simulink model "AMR_main_24a_TesteMobotic"  (R2024a)
settings: Solver=FixedStepAuto  StartTime=0.0  StopTime=inf  FixedStep=1e-3  RelTol=1e-3
model workspace (MAT data in the model file):
  RTK_health_condition = 30
  mdlWSDbList = ["tramontina_database_curtis.dbc" "tramontina_database_mobotic.dbc" "tramontina_database_nvidia.dbc" "tramontina_database_sick_modbus.dbc" "tramontina_database_xsens.dbc"]
undefined symbols (not defined in the file or in its folder): Down, Pull
libraries: tramontina_database_nvidialib x11, speedgoatlib_IO60X_IO69X x10, tramontina_database_curtislib x7, tramontina_database_xsenslib x4, tramontina_database_moboticlib x2, speedgoatlib_IO691 x2, canmsglib x1
(part 1 of 2)
settings Model: DataDictionary=configuration_dictionary.sldd  SimulationMode=external  ExtModeEnableFloating=off  ExtModeTrigDuration=100000  Creator=matlab.cut  LastModifiedBy=matlab.cut
settings SolverCC: ConcurrentTasks=on  PositivePriorityOrder=on
settings OptimizationCC: BlockReduction=off  DefaultParameterBehavior=Inlined  OptimizeBlockIOStorage=off  EnhancedBackFolding=on  PassReuseOutputArgsThreshold=0  OptimizeBlockOrder=speed  DifferentSizesBufferReuse=on
settings DebuggingCC: UnderspecifiedInitializationDetection=Classic  MergeDetectMultiDrivingBlocksExec=none  TasksWithSamePriorityMsg=none  ParameterTunabilityLossMsg=error
settings HardwareCC: ProdBitPerLong=64  ProdLongLongMode=on  ProdHWDeviceType=Intel->x86-64 (Linux 64)
settings ModelReferenceCC: PropagateSignalLabelsOutOfModel=off
settings SFSimCC: MATLABDynamicMemAlloc=off
settings RTWCC: Description=Speedgoat Real-Time Target Machine  SystemTargetFile=speedgoat.tlc  TemplateMakefile=slrealtime_default_tmf  Toolchain=Simulink Real-Time Toolchain  BuildConfiguration=Faster Runs  CodeExecutionProfiling=on  TargetLang=C++  GPUComputeCapability=3.5
settings CodeAppCC: ForceParamTrailComments=on  MaxIdLength=127  OperatorAnnotations=on
settings SimulinkRealTimeTargetCC: InstructionSetFMA=off  LogToMDFFile=off

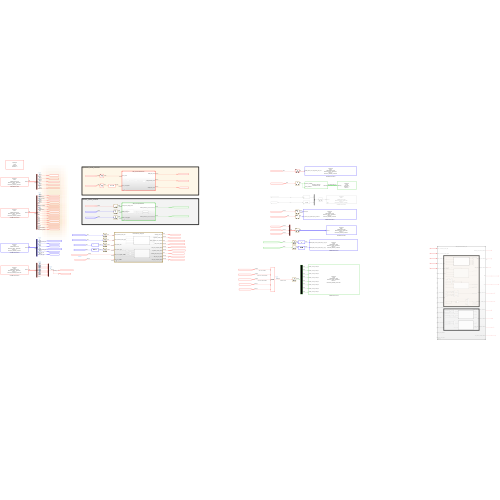
[thumbnail: Simulink's stored preview of the top-level diagram]
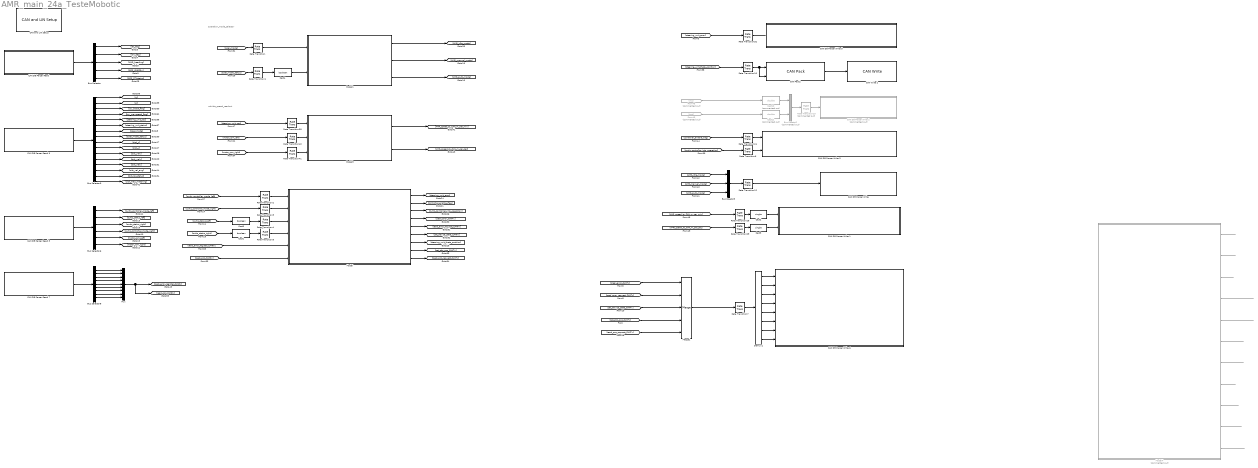
== system AMR_main_24a_TesteMobotic ==
  note: operation_mode_selector
  note: vehicle_speed_readout
  Bus Creator2 : BusCreator  Commented=on  Inputs=2
  Bus Creator3 : BusCreator  Inputs=3
  Bus Selector : BusSelector  OutputSignals=ID113_LongLat.latitude,ID113_LongLat.longitude,ID34_EulerAngles.yaw,ID17_StatusWord.GNSSfix,ID17_StatusWord.RtkStatus
  Bus Selector6 : BusSelector  OutputSignals=ID1830_controller_status_left.controller_mode_left,ID1830_controller_status_left.MessageStatus.Status,ID1831_controller_status_right.MessageStatus.Status,ID1831_controller_status_right.controller_mode_right,ID422_curtis_feedback_message_left.motor_rpm_left,ID423_curtis_feedback_message_right.motor_rpm_right
  Bus Selector8 : BusSelector  OutputSignals=ID1459_feedback_word.MessageStatus.Status,ID1459_feedback_word.byte0,ID1459_feedback_word.byte1,ID1459_feedback_word.byte2,ID1459_feedback_word.byte3,ID1459_feedback_word.byte4,ID1459_feedback_word.byte5,ID1459_feedback_word.byte6,ID1459_feedback_word.byte7
  Bus Selector9 : BusSelector  OutputSignals=ID368_joystick_axes.joystick_throttle,ID368_joystick_axes.joystick_direction,ID369_joystick_buttons.button_5,ID369_joystick_buttons.button_6,ID288_mobotic_feedback_pos.position_feedback,ID288_mobotic_feedback_pos.MessageStatus.Status,ID343_AMR_OperationMode.OperationMode,ID343_AMR_OperationMode.MessageStatus.Status,ID370_outdoor_scanner_PosX.X,ID371_outdoor_scanner_PosY.Y,ID372_outdoor_scanner_Yaw_Status.Yaw,ID373_outdoor_scanner_Odometer_Vel.velX,ID373_outdoor_scanner_Odometer_Vel.velY,ID373_outdoor_scanner_Odometer_Vel.velAng,ID372_outdoor_scanner_Yaw_Status.LocalizationStatus,ID372_outdoor_scanner_Yaw_Status.MapMatchingStatus
  CAN DB Parser Read : Subsystem
      settings: OpenFcn=sg_can.OpenFcnRead;
      mask Help: eval('sg.utils.help.show(''io_main/refentry_ref_can_ofa_parsing_read'');')
      mask Display: disp('Speedgoat\nIO691\nCAN DB Parser Read\nModule ID: IO691 - Module ID 1\nChannel:  1\ntramontina_database_xsens.dbc ');
  CAN DB Parser Read 3 : Subsystem
      settings: OpenFcn=sg_can.OpenFcnRead;
      mask Help: eval('sg.utils.help.show(''io_main/refentry_ref_can_ofa_parsing_read'');')
      mask Display: disp('Speedgoat\nIO691\nCAN DB Parser Read\nModule ID: IO691 - Module ID 1\nChannel:  1\ntramontina_database_curtis.dbc ');
  CAN DB Parser Read 7 : Subsystem
      settings: OpenFcn=sg_can.OpenFcnRead;
      mask Help: eval('sg.utils.help.show(''io_main/refentry_ref_can_ofa_parsing_read'');')
      mask Display: disp('Speedgoat\nIO691\nCAN DB Parser Read\nModule ID: IO691 - Module ID 1\nChannel:  1\ntramontina_database_mobotic.dbc ');
  CAN DB Parser Read 9 : Subsystem
      settings: OpenFcn=sg_can.OpenFcnRead;
      mask Help: eval('sg.utils.help.show(''io_main/refentry_ref_can_ofa_parsing_read'');')
      mask Display: disp('Speedgoat\nIO691\nCAN DB Parser Read\nModule ID: IO691 - Module ID 1\nChannel:  1\ntramontina_database_nvidia.dbc ');
  "CAN DB Parser Write " : Subsystem
      settings: OpenFcn=sg_can.OpenFcnWrite;
      mask Help: eval('sg.utils.help.show(''io_main/refentry_ref_can_ofa_parsing_write'');')
      mask Display: disp('Speedgoat\nIO691\nCAN DB Parser Write\nModule ID: IO691 - Module ID 1\nChannel:  1\ntramontina_database_nvidia.dbc ');
  CAN DB Parser Write 1 : Subsystem
      settings: OpenFcn=sg_can.OpenFcnWrite;
      mask Help: eval('sg.utils.help.show(''io_main/refentry_ref_can_ofa_parsing_write'');')
      mask Display: disp('Speedgoat\nIO691\nCAN DB Parser Write\nModule ID: IO691 - Module ID 1\nChannel:  1\ntramontina_database_nvidia.dbc ');
  CAN DB Parser Write 2 : Subsystem  Commented=on
      settings: OpenFcn=sg_can.OpenFcnWrite;
      mask Help: eval('sg.utils.help.show(''io_main/refentry_ref_can_ofa_parsing_write'');')
      mask Display: disp('Speedgoat\nIO691\nCAN DB Parser Write\nModule ID: IO691 - Module ID 1\nChannel:  1\ntramontina_database_curtis.dbc ');
  CAN DB Parser Write 3 : Subsystem
      settings: OpenFcn=sg_can.OpenFcnWrite;
      mask Help: eval('sg.utils.help.show(''io_main/refentry_ref_can_ofa_parsing_write'');')
      mask Display: disp('Speedgoat\nIO691\nCAN DB Parser Write\nModule ID: IO691 - Module ID 1\nChannel:  1\ntramontina_database_curtis.dbc ');
  CAN DB Parser Write 5 : Subsystem
      settings: OpenFcn=sg_can.OpenFcnWrite;
      mask Help: eval('sg.utils.help.show(''io_main/refentry_ref_can_ofa_parsing_write'');')
      mask Display: disp('Speedgoat\nIO691\nCAN DB Parser Write\nModule ID: IO691 - Module ID 1\nChannel:  1\ntramontina_database_nvidia.dbc ');
  CAN DB Parser Write 6 : Subsystem
      settings: OpenFcn=sg_can.OpenFcnWrite;
      mask Help: eval('sg.utils.help.show(''io_main/refentry_ref_can_ofa_parsing_write'');')
      mask Display: disp('Speedgoat\nIO691\nCAN DB Parser Write\nModule ID: IO691 - Module ID 1\nChannel:  1\ntramontina_database_mobotic.dbc ');
  CAN Pack2 : canmsglib/CAN Pack  MsgList=(none)  MsgName=CAN Msg  MsgIDType=Standard (11-bit identifier)  MsgIdentifier=0x120  MsgLength=8  Remote=off  ApplyMinMax=off  BusOutput=on  SignalInfo={ 'position_feedback', '0', '32', 'LE', 'signed', 'Standard', '0', '1', '0', '-inf', 'inf'; 'pulse_feedback', '32', '32', 'LE', 'signed', 'Standard', '0', '1', '0', '-Inf', 'Inf' }
      settings: DataFormat=manually specified signals
  CAN Write 2 : speedgoatlib_IO691/CAN Write   moduleType=IO691  id=1  channel=1  canType=CAN (HS)  messageType=CAN (HS)  useBusIn=on  numOfMsg=1  enableInput=off  enableStatusPort=off  ts=10e-3  initValues=[691 1 0.01 0 1 1 0 1 0 1]
      settings: SourceProductName=IO691
  "CAN and LIN Setup " : speedgoatlib_IO691/CAN and LIN Setup   moduleInitValues="[691    1    1   -1   -1]"  id=1  moduleType=IO691  pciSlot=-1  canChn1=CAN (HS)  canChn2=Disabled  canChn3=Disabled  canChn4=Disabled  linChn1=Disabled  linChn2=Disabled  canInitStructArray=[]  canTermStructArray=[]  gpioChnx=Disabled  canChn1InitValues="[2   2   8   1  16   3  19   2   2   5   2   0]"  arbBdrChn1=500 kBaud  clockDividerChn1=Enable  arbManBdrChn1=[8,1,16,3]  fdBdrChn1=5.0 MBaud  fdManBdrChn1=[2,2,5,2]  termResistor1=off  canChn2InitValues="[1   0   2   8  31   8  19   2   2   5   2   0]"  arbBdrChn2=1.0 MBaud  clockDividerChn2=Enable  arbManBdrChn2=[2,8,31,8]  fdBdrChn2=5.0 MBaud  fdManBdrChn2=[2,2,5,2]  termResistor2=off  canChn3InitValues="[1   0   2   8  31   8  19   2   2   5   2   0]"  arbBdrChn3=1.0 MBaud  clockDividerChn3=Enable  arbManBdrChn3=[2,8,31,8]  fdBdrChn3=5.0 MBaud  fdManBdrChn3=[2,2,5,2]  termResistor3=off  canChn4InitValues="[1   0   2   8  31   8  19   2   2   5   2   0]"  arbBdrChn4=1.0 MBaud  clockDividerChn4=Enable  arbManBdrChn4=[2,8,31,8]  fdBdrChn4=5.0 MBaud  fdManBdrChn4=[2,2,5,2]  termResistor4=off  linChn1InitValues="[0  9600]"  linBtrChn1=9600  linChn2InitValues="[0  9600]"  linBtrChn2=9600  doInitTermStruct="[0  5  0  0  0]"  parDoChannels=[1 2]  parDoVoltage=5  parDoInitValues=0  parDoReset=1  parNumOfDoS=0  parDiChannels=[3 4]  parDiVoltage=5  parDiPull=Pull-Down
      settings: LibrarySourceBlock=speedgoatlib_IO602_IO691/CAN and LIN Setup
  Cast1 : DataTypeConversion  OutDataTypeStr=boolean  SaturateOnIntegerOverflow=off  RndMeth=Floor
  Cast10 : DataTypeConversion  Commented=on  OutDataTypeStr=double  SaturateOnIntegerOverflow=off  RndMeth=Floor
  Cast11 : DataTypeConversion  Commented=on  OutDataTypeStr=double  SaturateOnIntegerOverflow=off  RndMeth=Floor
  Cast2 : DataTypeConversion  OutDataTypeStr=single  SaturateOnIntegerOverflow=off  RndMeth=Floor
  Cast3 : DataTypeConversion  OutDataTypeStr=single  SaturateOnIntegerOverflow=off  RndMeth=Floor
  Cast4 : DataTypeConversion  OutDataTypeStr=boolean  SaturateOnIntegerOverflow=off  RndMeth=Floor
  Cast5 : DataTypeConversion  OutDataTypeStr=boolean  SaturateOnIntegerOverflow=off  RndMeth=Floor
  Demux1 : Demux  Outputs=8
  From43 : From  Commented=on  GotoTag=rws
  From45 : From  Commented=on  GotoTag=lws
  Merge1 : Merge  Inputs=5
  Model : ModelReference  ModelNameDialog=MoboticStartup_TimingSync.slx  SimulationMode=Normal  ModelReferenceVersion=1.12
  Model1 : ModelReference  ModelNameDialog=AMR_OperationModeSelector.slx  SimulationMode=Normal  ModelReferenceVersion=2.2
  Model3 : ModelReference  ModelNameDialog=AMR_VehicleSpeedReadout.slx  SimulationMode=Normal  ModelReferenceVersion=2.1
  Model4 : ModelReference  Commented=on  ModelNameDialog=AMR_MotorControlUnit_23b.slx  SimulationMode=Normal  ModelReferenceVersion=2.8
  Mux : Mux  Inputs=9
  Rate Transition{,1..7,10,24,28..29,32,38,40..41} (16 alike) : RateTransition
  Rate Transition12 : RateTransition  Deterministic=off
  Rate Transition15 : RateTransition  Commented=on
  wires:
  Rate Transition32/1 -> ?
  Rate Transition28/1 -> Cast2/1
  [AMR_speed_to_CAN_m_per_sec] -> Rate Transition29/1
  [AMR_speed_to_CAN_m_per_min] -> Rate Transition28/1
  CAN Pack2/1 -> CAN Write 2/1
  Bus Creator2/1 -> Rate Transition15/1
  From43/1 -> Cast11/1  "rws"
  Cast10/1 -> Bus Creator2/1
  Rate Transition6/1 -> CAN DB Parser Write 3/2(ID0_curtis_input_operational.pre_operational)
  Bus Creator3/1 -> Rate Transition12/1
  [steering_unit_error] -> Rate Transition32/1
  Rate Transition10/1 -> CAN Pack2/2, CAN Pack2/1
  Rate Transition29/1 -> Cast3/1
  [curtis_controller_into_operation] -> Rate Transition6/1
  From45/1 -> Cast10/1  "lws"
  Cast11/1 -> Bus Creator2/2
  [steering_unit_theta_position] -> Rate Transition10/1
  [controller_enable_flag] -> Rate Transition24/1
  Rate Transition15/1 -> CAN DB Parser Write 2/1(CAN Tx)
  Rate Transition24/1 -> CAN DB Parser Write 3/1(Enable Input)
  [oper_mode] -> Rate Transition/1
  Cast4/1 -> Model1/2
  Model1/1 -> [AMR_idle_mode]
  Model1/2 -> [AMR_manual_mode]
  Model1/3 -> [AMR_auto_mode]
  ? -> Model4/3
  ? -> Model4/1
  ? -> Model4/4
  ? -> Model4/2
  [motor_rpm_right] -> Rate Transition41/1
  [steering_unit_pos] -> Rate Transition38/1
  [motor_rpm_left] -> Rate Transition40/1
  Model3/1 -> [AMR_speed_to_CAN_m_per_min]
  Model3/2 -> [AMR_speed_to_CAN_m_per_sec]
  Rate Transition38/1 -> Model3/1
  Rate Transition41/1 -> Model3/3
  Rate Transition40/1 -> Model3/2
  Cast2/1 -> CAN DB Parser Write 1/1(ID290_AMR_vehicle_speed.speed_m_per_min)
  Cast3/1 -> CAN DB Parser Write 1/2(ID290_AMR_vehicle_speed.speed_m_per_s)
  [oper_mode_status] -> Rate Transition1/1
  [AMR_idle_mode] -> Bus Creator3/1
  [AMR_auto_mode] -> Bus Creator3/3
  [AMR_manual_mode] -> Bus Creator3/2
  Rate Transition12/1 -> "CAN DB Parser Write "/1(CAN Tx)
  Rate Transition/1 -> Model1/1
  Rate Transition1/1 -> Cast4/1
  Model4/1 -> ?
  Model4/5 -> ?
  Model4/4 -> ?
  Model4/6 -> ?
  Model4/7 -> ?
  Model4/8 -> ?
  Model4/2 -> ?  "lws"
  Model4/3 -> ?  "rws"
  Model4/9 -> ?
  Model4/10 -> ?
  Model4/11 -> ?
  Bus Selector/1 -> [lat_deg]  "<latitude>"
  Bus Selector6/2 -> [curtis_status_left]  "<Status>"
  Bus Selector9/8 -> [oper_mode_status]  "<Status>"
  Bus Selector9/7 -> [oper_mode]  "<OperationMode>"
  Bus Selector9/3 -> [joy_boost_flag]  "<button_5>"
  Bus Selector9/1 -> [xj]  "<joystick_throttle>"
  Bus Selector9/4 -> [joy_maxspeed_flag]  "<button_6>"
  Bus Selector/4 -> [GPS_GNSSfix]  "<GNSSfix>"
  Bus Selector9/2 -> [yj]  "<joystick_direction>"
  Bus Selector8/7 -> Mux/7  "<byte5>"
  CAN DB Parser Read 9/1(CAN Rx) -> Bus Selector9/1
  Bus Selector8/5 -> Mux/5  "<byte3>"
  Bus Selector9/13 -> [sick_vely]  "<velY>"
  Bus Selector8/1 -> Mux/1  "<Status>"
  Bus Selector9/5 -> [steering_unit_pos]  "<position_feedback>"
  Bus Selector8/2 -> Mux/2  "<byte0>"
  CAN DB Parser Read 3/1(CAN Rx) -> Bus Selector6/1
  Bus Selector9/9 -> [sick_x]  "<X>"
  CAN DB Parser Read 7/1(CAN Rx) -> Bus Selector8/1
  Bus Selector8/3 -> Mux/3  "<byte1>"
  Bus Selector8/6 -> Mux/6  "<byte4>"
  Mux/1 -> [read_pos_CANRx], [read_error_register_CANRx]  "mobotic_Rx"
  Bus Selector8/8 -> Mux/8  "<byte6>"
  Bus Selector8/9 -> Mux/9  "<byte7>"
  Bus Selector6/4 -> [curtis_controller_mode_right]  "<controller_mode_right>"
  Bus Selector9/10 -> [sick_y]  "<Y>"
  Bus Selector9/16 -> [sick_map_matching]  "<MapMatchingStatus>"
  Bus Selector9/12 -> [sick_velx]  "<velX>"
  Bus Selector9/15 -> [sick_loc_status]  "<LocalizationStatus>"
  Bus Selector/5 -> [GPS_RTKstatus]  "<RtkStatus>"
  Bus Selector9/14 -> [sick_vel_ang]  "<velAng>"
  Bus Selector9/6 -> [steering_unit_status]  "<Status>"
  Bus Selector6/5 -> [motor_rpm_left]  "<motor_rpm_left>"
  Bus Selector9/11 -> [sick_yaw]  "<Yaw>"
  Bus Selector6/6 -> [motor_rpm_right]  "<motor_rpm_right>"
  Bus Selector/3 -> [AMR_heading]  "<yaw>"
  Bus Selector6/3 -> [curtis_status_right]  "<Status>"
  Bus Selector8/4 -> Mux/4  "<byte2>"
  Bus Selector6/1 -> [curtis_controller_mode_left]  "<controller_mode_left>"
  CAN DB Parser Read/1(CAN Rx) -> Bus Selector/1
  Bus Selector/2 -> [lon_deg]  "<longitude>"
  ? -> Model4/5
  [curtis_controller_mode_left] -> Rate Transition2/1
  Cast5/1 -> Rate Transition4/1
  Cast1/1 -> Rate Transition5/1
  [curtis_controller_mode_right] -> Rate Transition3/1
  [curtis_status_left] -> Cast5/1
  [curtis_status_right] -> Cast1/1
  [read_error_register_CANRx] -> Model/5
  [read_pos_CANRx] -> Model/6
  Model/9 -> [read_pos_request_CANTx]
  Model/8 -> [set_abs_pos_CANTx]
  Model/7 -> [steering_unit_theta_position]
  Model/5 -> [read_error_request_CANTx]
  Model/6 -> [set_device_state_CANTx]
  Model/4 -> [clear_error_CANTx]
  Model/3 -> [curtis_controller_into_operation]
  Model/2 -> [controller_enable_flag]
  Model/1 -> [steering_unit_error]
  [clear_error_CANTx] -> Merge1/1  "clear_error_CANTx"
  Merge1/1 -> Rate Transition7/1  "mobotic_merge"
  [read_error_request_CANTx] -> Merge1/2  "read_error_request_CANTx"
  [set_device_state_CANTx] -> Merge1/3  "set_device_state_CANTx"
  [set_abs_pos_CANTx] -> Merge1/4
  [read_pos_request_CANTx] -> Merge1/5
  Rate Transition2/1 -> Model/1
  Rate Transition3/1 -> Model/2
  Rate Transition4/1 -> Model/3
  Rate Transition5/1 -> Model/4
  Rate Transition7/1 -> Demux1/1
  Demux1/1 -> CAN DB Parser Write 6/1(ID1587_control_word.byte0)
  Demux1/2 -> CAN DB Parser Write 6/2(ID1587_control_word.byte1)
  Demux1/3 -> CAN DB Parser Write 6/3(ID1587_control_word.byte2)
  Demux1/4 -> CAN DB Parser Write 6/4(ID1587_control_word.byte3)
  Demux1/5 -> CAN DB Parser Write 6/5(ID1587_control_word.byte4)
  Demux1/6 -> CAN DB Parser Write 6/6(ID1587_control_word.byte5)
  Demux1/7 -> CAN DB Parser Write 6/7(ID1587_control_word.byte6)
  Demux1/8 -> CAN DB Parser Write 6/8(ID1587_control_word.byte7)

== system AMR_main_24a_TesteMobotic/CAN DB Parser Read ==
  ReadSubsystem : Subsystem
  UnpackSubsystem : Subsystem
  CAN Rx : Outport
  wires:
  ReadSubsystem/1(Raw_Rx) -> UnpackSubsystem/1(Unpack_In)
  ReadSubsystem/2(Status_Rx) -> UnpackSubsystem/2(Status Inport)
  UnpackSubsystem/1(Unpack_Out) -> CAN Rx/1

== system AMR_main_24a_TesteMobotic/CAN DB Parser Read 3 ==
  ReadSubsystem : Subsystem
  UnpackSubsystem : Subsystem
  CAN Rx : Outport
  wires:
  ReadSubsystem/1(Raw_Rx) -> UnpackSubsystem/1(Unpack_In)
  ReadSubsystem/2(Status_Rx) -> UnpackSubsystem/2(Status Inport)
  UnpackSubsystem/1(Unpack_Out) -> CAN Rx/1

== system AMR_main_24a_TesteMobotic/CAN DB Parser Read 7 ==
  ReadSubsystem : Subsystem
  UnpackSubsystem : Subsystem
  CAN Rx : Outport
  wires:
  ReadSubsystem/1(Raw_Rx) -> UnpackSubsystem/1(Unpack_In)
  ReadSubsystem/2(Status_Rx) -> UnpackSubsystem/2(Status Inport)
  UnpackSubsystem/1(Unpack_Out) -> CAN Rx/1

== system AMR_main_24a_TesteMobotic/CAN DB Parser Read 9 ==
  ReadSubsystem : Subsystem
  UnpackSubsystem : Subsystem
  CAN Rx : Outport
  wires:
  ReadSubsystem/1(Raw_Rx) -> UnpackSubsystem/1(Unpack_In)
  ReadSubsystem/2(Status_Rx) -> UnpackSubsystem/2(Status Inport)
  UnpackSubsystem/1(Unpack_Out) -> CAN Rx/1

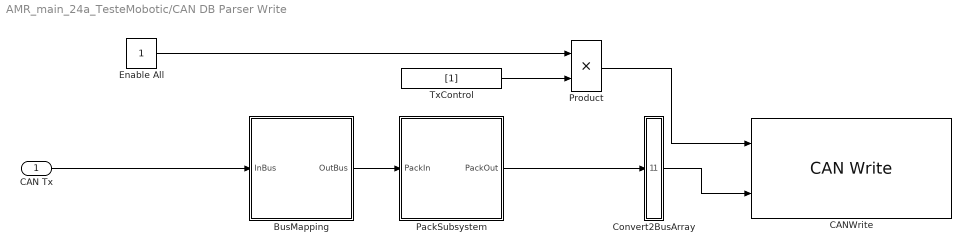
== system AMR_main_24a_TesteMobotic/CAN DB Parser Write  ==
  CAN Tx : Inport
  BusMapping : Subsystem
  CANWrite : speedgoatlib_IO60X_IO69X/CAN/CAN Write   moduleType=IO691  id=1  channel=1  canType=CAN (HS)  messageType=CAN (HS)  useBusIn=on  numOfMsg=1  enableInput=on  enableStatusPort=off  ts=500e-3  initValues=[691 1 0.5 0 1 1 0 1 1 1]
  Convert2BusArray : Subsystem
  Enable All : Constant  OutDataTypeStr=boolean
  PackSubsystem : Subsystem
  Product : Product  OutDataTypeStr=uint32
  TxControl : Constant  Value=[1]  OutDataTypeStr=uint32
  wires:
  PackSubsystem/1(PackOut) -> Convert2BusArray/1(InBus)
  Convert2BusArray/1(BusArrayOut) -> CANWrite/2
  Product/1 -> CANWrite/1
  TxControl/1 -> Product/2
  Enable All/1 -> Product/1
  CAN Tx/1 -> BusMapping/1(InBus)
  BusMapping/1(OutBus) -> PackSubsystem/1(PackIn)

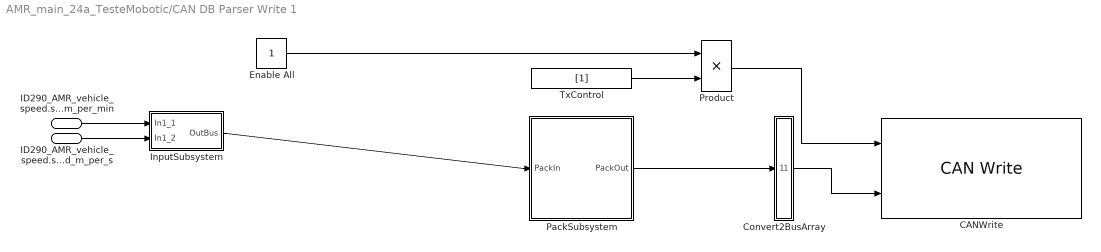
== system AMR_main_24a_TesteMobotic/CAN DB Parser Write 1 ==
  ID290_AMR_vehicle_speed.speed_m_per_min : Inport
  ID290_AMR_vehicle_speed.speed_m_per_s : Inport  Port=2
  CANWrite : speedgoatlib_IO60X_IO69X/CAN/CAN Write   moduleType=IO691  id=1  channel=1  canType=CAN (HS)  messageType=CAN (HS)  useBusIn=on  numOfMsg=1  enableInput=on  enableStatusPort=off  ts=50e-3  initValues=[691 1 0.05 0 1 1 0 1 1 1]
  Convert2BusArray : Subsystem
  Enable All : Constant  OutDataTypeStr=boolean
  InputSubsystem : Subsystem
  PackSubsystem : Subsystem
  Product : Product  OutDataTypeStr=uint32
  TxControl : Constant  Value=[1]  OutDataTypeStr=uint32
  wires:
  PackSubsystem/1(PackOut) -> Convert2BusArray/1(InBus)
  Convert2BusArray/1(BusArrayOut) -> CANWrite/2
  Product/1 -> CANWrite/1
  TxControl/1 -> Product/2
  Enable All/1 -> Product/1
  ID290_AMR_vehicle_speed.speed_m_per_min/1 -> InputSubsystem/1(In1_1)
  ID290_AMR_vehicle_speed.speed_m_per_s/1 -> InputSubsystem/2(In1_2)
  InputSubsystem/1(OutBus) -> PackSubsystem/1(PackIn)

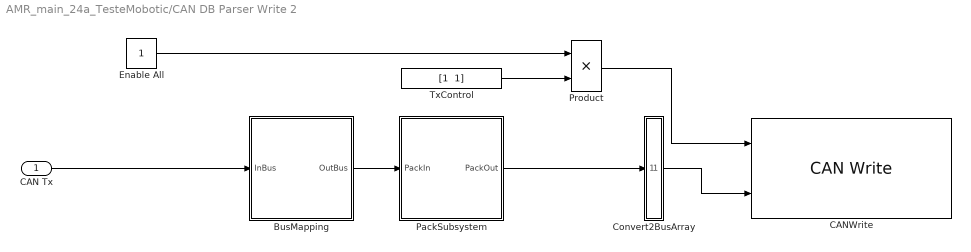
== system AMR_main_24a_TesteMobotic/CAN DB Parser Write 2 ==
  CAN Tx : Inport
  BusMapping : Subsystem
  CANWrite : speedgoatlib_IO60X_IO69X/CAN/CAN Write   moduleType=IO691  id=1  channel=1  canType=CAN (HS)  messageType=CAN (HS)  useBusIn=on  numOfMsg=2  enableInput=on  enableStatusPort=off  ts=10e-3  initValues=[691 1 0.01 0 1 1 0 2 1 1]
  Convert2BusArray : Subsystem
  Enable All : Constant  OutDataTypeStr=boolean
  PackSubsystem : Subsystem
  Product : Product  OutDataTypeStr=uint32
  TxControl : Constant  Value="[1  1]"  OutDataTypeStr=uint32
  wires:
  PackSubsystem/1(PackOut) -> Convert2BusArray/1(InBus)
  Convert2BusArray/1(BusArrayOut) -> CANWrite/2
  Product/1 -> CANWrite/1
  TxControl/1 -> Product/2
  Enable All/1 -> Product/1
  CAN Tx/1 -> BusMapping/1(InBus)
  BusMapping/1(OutBus) -> PackSubsystem/1(PackIn)

== system AMR_main_24a_TesteMobotic/CAN DB Parser Write 3 ==
  Enable Input : Inport  OutDataTypeStr=boolean
  ID0_curtis_input_operational.pre_operational : Inport  Port=2
  CANWrite : speedgoatlib_IO60X_IO69X/CAN/CAN Write   moduleType=IO691  id=1  channel=1  canType=CAN (HS)  messageType=CAN (HS)  useBusIn=on  numOfMsg=1  enableInput=on  enableStatusPort=off  ts=500e-3  initValues=[691 1 0.5 0 1 1 0 1 1 1]
  Convert2BusArray : Subsystem
  InputSubsystem : Subsystem
  PackSubsystem : Subsystem
  Product : Product  OutDataTypeStr=uint32
  TxControl : Constant  Value=[1]  OutDataTypeStr=uint32
  wires:
  PackSubsystem/1(PackOut) -> Convert2BusArray/1(InBus)
  Convert2BusArray/1(BusArrayOut) -> CANWrite/2
  Product/1 -> CANWrite/1
  TxControl/1 -> Product/2
  Enable Input/1 -> Product/1
  ID0_curtis_input_operational.pre_operational/1 -> InputSubsystem/1(In1_1)
  InputSubsystem/1(OutBus) -> PackSubsystem/1(PackIn)

== system AMR_main_24a_TesteMobotic/CAN DB Parser Write 5 ==
  ID289_mobotic_error_flag.steering_unit_error : Inport
  CANWrite : speedgoatlib_IO60X_IO69X/CAN/CAN Write   moduleType=IO691  id=1  channel=1  canType=CAN (HS)  messageType=CAN (HS)  useBusIn=on  numOfMsg=1  enableInput=on  enableStatusPort=off  ts=500e-3  initValues=[691 1 0.5 0 1 1 0 1 1 1]
  Convert2BusArray : Subsystem
  Enable All : Constant  OutDataTypeStr=boolean
  InputSubsystem : Subsystem
  PackSubsystem : Subsystem
  Product : Product  OutDataTypeStr=uint32
  TxControl : Constant  Value=[1]  OutDataTypeStr=uint32
  wires:
  PackSubsystem/1(PackOut) -> Convert2BusArray/1(InBus)
  Convert2BusArray/1(BusArrayOut) -> CANWrite/2
  Product/1 -> CANWrite/1
  TxControl/1 -> Product/2
  Enable All/1 -> Product/1
  ID289_mobotic_error_flag.steering_unit_error/1 -> InputSubsystem/1(In1_1)
  InputSubsystem/1(OutBus) -> PackSubsystem/1(PackIn)

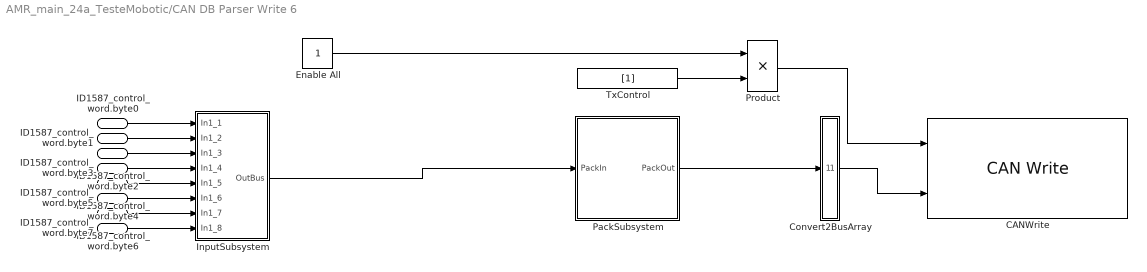
== system AMR_main_24a_TesteMobotic/CAN DB Parser Write 6 ==
  ID1587_control_word.byte0 : Inport
  ID1587_control_word.byte1 : Inport  Port=2
  ID1587_control_word.byte2 : Inport  Port=3
  ID1587_control_word.byte3 : Inport  Port=4
  ID1587_control_word.byte4 : Inport  Port=5
  ID1587_control_word.byte5 : Inport  Port=6
  ID1587_control_word.byte6 : Inport  Port=7
  ID1587_control_word.byte7 : Inport  Port=8
  CANWrite : speedgoatlib_IO60X_IO69X/CAN/CAN Write   moduleType=IO691  id=1  channel=1  canType=CAN (HS)  messageType=CAN (HS)  useBusIn=on  numOfMsg=1  enableInput=on  enableStatusPort=off  ts=10e-3  initValues=[691 1 0.01 0 1 1 0 1 1 1]
  Convert2BusArray : Subsystem
  Enable All : Constant  OutDataTypeStr=boolean
  InputSubsystem : Subsystem
  PackSubsystem : Subsystem
  Product : Product  OutDataTypeStr=uint32
  TxControl : Constant  Value=[1]  OutDataTypeStr=uint32
  wires:
  PackSubsystem/1(PackOut) -> Convert2BusArray/1(InBus)
  Convert2BusArray/1(BusArrayOut) -> CANWrite/2
  Product/1 -> CANWrite/1
  TxControl/1 -> Product/2
  Enable All/1 -> Product/1
  ID1587_control_word.byte0/1 -> InputSubsystem/1(In1_1)
  ID1587_control_word.byte1/1 -> InputSubsystem/2(In1_2)
  ID1587_control_word.byte2/1 -> InputSubsystem/3(In1_3)
  ID1587_control_word.byte3/1 -> InputSubsystem/4(In1_4)
  ID1587_control_word.byte4/1 -> InputSubsystem/5(In1_5)
  ID1587_control_word.byte5/1 -> InputSubsystem/6(In1_6)
  ID1587_control_word.byte6/1 -> InputSubsystem/7(In1_7)
  ID1587_control_word.byte7/1 -> InputSubsystem/8(In1_8)
  InputSubsystem/1(OutBus) -> PackSubsystem/1(PackIn)

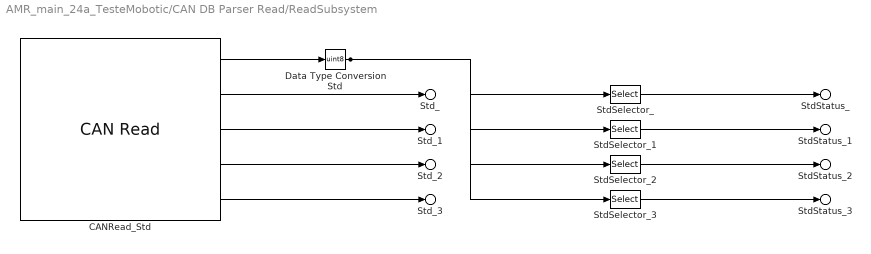
== system AMR_main_24a_TesteMobotic/CAN DB Parser Read/ReadSubsystem ==
  CANRead_Std : speedgoatlib_IO60X_IO69X/CAN/CAN Read   moduleType=IO691  id=1  channel=1  canType=CAN (HS)  messageType=CAN (HS)  useBusOut=on  HasMulRead=Specify by IDs  MsgIDlist="[17   34  113  118]"  isEFF=off  LabelInHex=off  enableInput=off  initValues=[691 1 -1 0 1 1 0 1 2 0 4 17 34 113 118]  ts=-1
  Data Type ConversionStd : DataTypeConversion  OutDataTypeStr=uint8  SaturateOnIntegerOverflow=off  RndMeth=Floor
  StdSelector_ : Selector  IndexOptions=Index vector (dialog)  Indices=1  OutputSizes=1
  StdSelector_1 : Selector  IndexOptions=Index vector (dialog)  Indices=2  OutputSizes=1
  StdSelector_2 : Selector  IndexOptions=Index vector (dialog)  Indices=3  OutputSizes=1
  StdSelector_3 : Selector  IndexOptions=Index vector (dialog)  Indices=4  OutputSizes=1
  Std_ : Outport  PortName=Raw_Rx  Element=Std.ID17
  Std_1 : Outport  PortName=Raw_Rx  Element=Std.ID34
  Std_2 : Outport  PortName=Raw_Rx  Element=Std.ID113
  Std_3 : Outport  PortName=Raw_Rx  Element=Std.ID118
  StdStatus_ : Outport  Port=2  PortName=Status_Rx  Element=Std.ID17
  StdStatus_1 : Outport  Port=2  PortName=Status_Rx  Element=Std.ID34
  StdStatus_2 : Outport  Port=2  PortName=Status_Rx  Element=Std.ID113
  StdStatus_3 : Outport  Port=2  PortName=Status_Rx  Element=Std.ID118
  wires:
  CANRead_Std/1 -> Data Type ConversionStd/1
  CANRead_Std/2 -> Std_/1
  CANRead_Std/3 -> Std_1/1
  CANRead_Std/4 -> Std_2/1
  CANRead_Std/5 -> Std_3/1
  Data Type ConversionStd/1 -> StdSelector_/1, StdSelector_1/1, StdSelector_2/1, StdSelector_3/1
  StdSelector_/1 -> StdStatus_/1
  StdSelector_1/1 -> StdStatus_1/1
  StdSelector_2/1 -> StdStatus_2/1
  StdSelector_3/1 -> StdStatus_3/1

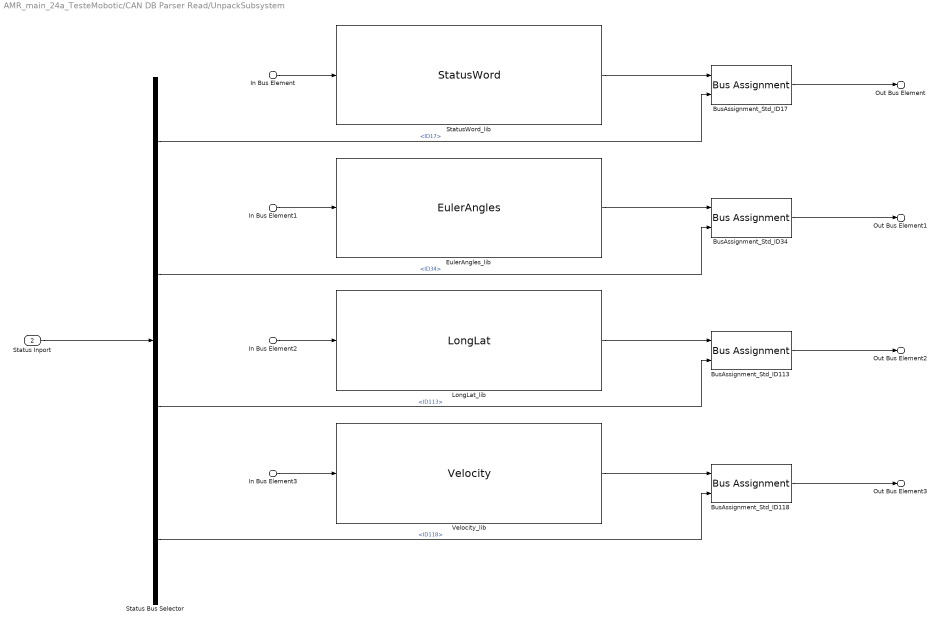
== system AMR_main_24a_TesteMobotic/CAN DB Parser Read/UnpackSubsystem ==
  In Bus Element : Inport  PortName=Unpack_In  Element=Std.ID17
  In Bus Element1 : Inport  PortName=Unpack_In  Element=Std.ID34
  In Bus Element2 : Inport  PortName=Unpack_In  Element=Std.ID113
  In Bus Element3 : Inport  PortName=Unpack_In  Element=Std.ID118
  Status Inport : Inport  Port=2
  BusAssignment_Std_ID{17,34,113,118} (4 alike) : BusAssignment  AssignedSignals=MessageStatus.Status
  EulerAngles_lib : tramontina_database_xsenslib/CAN unpack/EulerAngles  SystemSampleTime=-1  VariantActivationTime=update diagram  AllowFlexibleInterface=on  Latency=0  AutoFrameSizeCalculation=off
  LongLat_lib : tramontina_database_xsenslib/CAN unpack/LongLat  SystemSampleTime=-1  VariantActivationTime=update diagram  AllowFlexibleInterface=on  Latency=0  AutoFrameSizeCalculation=off
  Status Bus Selector : BusSelector  OutputSignals=Std.ID17,Std.ID34,Std.ID113,Std.ID118
  StatusWord_lib : tramontina_database_xsenslib/CAN unpack/StatusWord  SystemSampleTime=-1  VariantActivationTime=update diagram  AllowFlexibleInterface=on  Latency=0  AutoFrameSizeCalculation=off
  Velocity_lib : tramontina_database_xsenslib/CAN unpack/Velocity  SystemSampleTime=-1  VariantActivationTime=update diagram  AllowFlexibleInterface=on  Latency=0  AutoFrameSizeCalculation=off
  Out Bus Element : Outport  PortName=Unpack_Out  Element=ID17_StatusWord
  Out Bus Element1 : Outport  PortName=Unpack_Out  Element=ID34_EulerAngles
  Out Bus Element2 : Outport  PortName=Unpack_Out  Element=ID113_LongLat
  Out Bus Element3 : Outport  PortName=Unpack_Out  Element=ID118_Velocity
  wires:
  In Bus Element/1 -> StatusWord_lib/1
  StatusWord_lib/1 -> BusAssignment_Std_ID17/1
  BusAssignment_Std_ID17/1 -> Out Bus Element/1
  In Bus Element1/1 -> EulerAngles_lib/1
  EulerAngles_lib/1 -> BusAssignment_Std_ID34/1
  BusAssignment_Std_ID34/1 -> Out Bus Element1/1
  In Bus Element2/1 -> LongLat_lib/1
  LongLat_lib/1 -> BusAssignment_Std_ID113/1
  BusAssignment_Std_ID113/1 -> Out Bus Element2/1
  In Bus Element3/1 -> Velocity_lib/1
  Velocity_lib/1 -> BusAssignment_Std_ID118/1
  BusAssignment_Std_ID118/1 -> Out Bus Element3/1
  Status Inport/1 -> Status Bus Selector/1
  Status Bus Selector/1 -> BusAssignment_Std_ID17/2  "<ID17>"
  Status Bus Selector/2 -> BusAssignment_Std_ID34/2  "<ID34>"
  Status Bus Selector/3 -> BusAssignment_Std_ID113/2  "<ID113>"
  Status Bus Selector/4 -> BusAssignment_Std_ID118/2  "<ID118>"

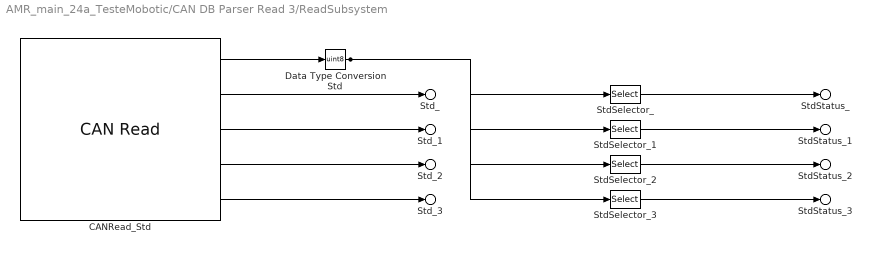
== system AMR_main_24a_TesteMobotic/CAN DB Parser Read 3/ReadSubsystem ==
  CANRead_Std : speedgoatlib_IO60X_IO69X/CAN/CAN Read   moduleType=IO691  id=1  channel=1  canType=CAN (HS)  messageType=CAN (HS)  useBusOut=on  HasMulRead=Specify by IDs  MsgIDlist="[422   423  1830  1831]"  isEFF=off  LabelInHex=off  enableInput=off  initValues=[691 1 0.05 0 1 1 0 1 2 0 4 422 423 1830 1831]  ts=50e-3
  Data Type ConversionStd : DataTypeConversion  OutDataTypeStr=uint8  SaturateOnIntegerOverflow=off  RndMeth=Floor
  StdSelector_ : Selector  IndexOptions=Index vector (dialog)  Indices=1  OutputSizes=1
  StdSelector_1 : Selector  IndexOptions=Index vector (dialog)  Indices=2  OutputSizes=1
  StdSelector_2 : Selector  IndexOptions=Index vector (dialog)  Indices=3  OutputSizes=1
  StdSelector_3 : Selector  IndexOptions=Index vector (dialog)  Indices=4  OutputSizes=1
  Std_ : Outport  PortName=Raw_Rx  Element=Std.ID422
  Std_1 : Outport  PortName=Raw_Rx  Element=Std.ID423
  Std_2 : Outport  PortName=Raw_Rx  Element=Std.ID1830
  Std_3 : Outport  PortName=Raw_Rx  Element=Std.ID1831
  StdStatus_ : Outport  Port=2  PortName=Status_Rx  Element=Std.ID422
  StdStatus_1 : Outport  Port=2  PortName=Status_Rx  Element=Std.ID423
  StdStatus_2 : Outport  Port=2  PortName=Status_Rx  Element=Std.ID1830
  StdStatus_3 : Outport  Port=2  PortName=Status_Rx  Element=Std.ID1831
  wires:
  CANRead_Std/1 -> Data Type ConversionStd/1
  CANRead_Std/2 -> Std_/1
  CANRead_Std/3 -> Std_1/1
  CANRead_Std/4 -> Std_2/1
  CANRead_Std/5 -> Std_3/1
  Data Type ConversionStd/1 -> StdSelector_/1, StdSelector_1/1, StdSelector_2/1, StdSelector_3/1
  StdSelector_/1 -> StdStatus_/1
  StdSelector_1/1 -> StdStatus_1/1
  StdSelector_2/1 -> StdStatus_2/1
  StdSelector_3/1 -> StdStatus_3/1

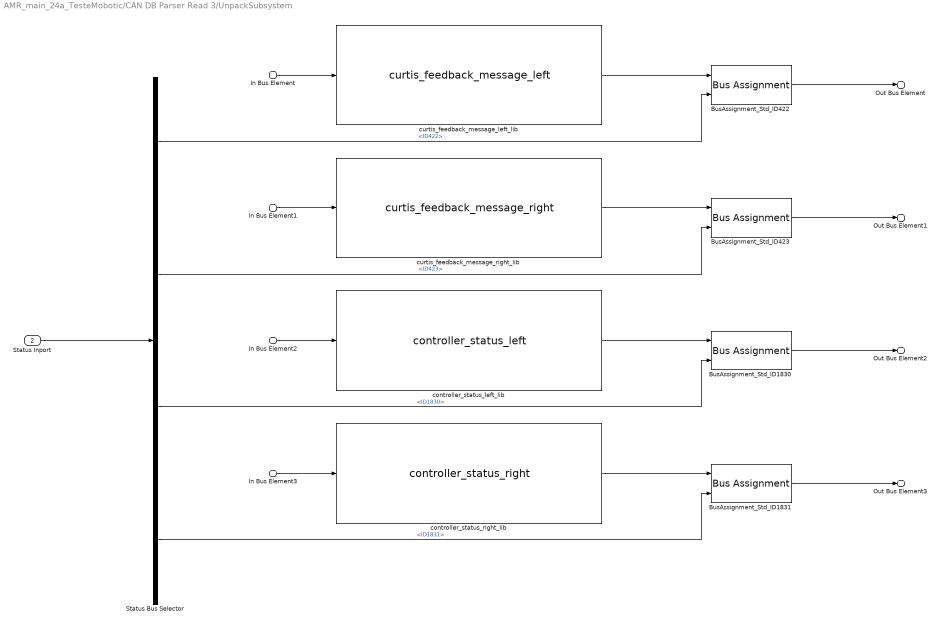
== system AMR_main_24a_TesteMobotic/CAN DB Parser Read 3/UnpackSubsystem ==
  In Bus Element : Inport  PortName=Unpack_In  Element=Std.ID422
  In Bus Element1 : Inport  PortName=Unpack_In  Element=Std.ID423
  In Bus Element2 : Inport  PortName=Unpack_In  Element=Std.ID1830
  In Bus Element3 : Inport  PortName=Unpack_In  Element=Std.ID1831
  Status Inport : Inport  Port=2
  BusAssignment_Std_ID{422..423,1830..1831} (4 alike) : BusAssignment  AssignedSignals=MessageStatus.Status
  Status Bus Selector : BusSelector  OutputSignals=Std.ID422,Std.ID423,Std.ID1830,Std.ID1831
  controller_status_left_lib : tramontina_database_curtislib/CAN unpack/controller_status_left  SystemSampleTime=-1  VariantActivationTime=update diagram  AllowFlexibleInterface=on  Latency=0  AutoFrameSizeCalculation=off
  controller_status_right_lib : tramontina_database_curtislib/CAN unpack/controller_status_right  SystemSampleTime=-1  VariantActivationTime=update diagram  AllowFlexibleInterface=on  Latency=0  AutoFrameSizeCalculation=off
  curtis_feedback_message_left_lib : tramontina_database_curtislib/CAN unpack/curtis_feedback_message_left  SystemSampleTime=-1  VariantActivationTime=update diagram  AllowFlexibleInterface=on  Latency=0  AutoFrameSizeCalculation=off
  curtis_feedback_message_right_lib : tramontina_database_curtislib/CAN unpack/curtis_feedback_message_right  SystemSampleTime=-1  VariantActivationTime=update diagram  AllowFlexibleInterface=on  Latency=0  AutoFrameSizeCalculation=off
  Out Bus Element : Outport  PortName=Unpack_Out  Element=ID422_curtis_feedback_message_left
  Out Bus Element1 : Outport  PortName=Unpack_Out  Element=ID423_curtis_feedback_message_right
  Out Bus Element2 : Outport  PortName=Unpack_Out  Element=ID1830_controller_status_left
  Out Bus Element3 : Outport  PortName=Unpack_Out  Element=ID1831_controller_status_right
  wires:
  In Bus Element/1 -> curtis_feedback_message_left_lib/1
  curtis_feedback_message_left_lib/1 -> BusAssignment_Std_ID422/1
  BusAssignment_Std_ID422/1 -> Out Bus Element/1
  In Bus Element1/1 -> curtis_feedback_message_right_lib/1
  curtis_feedback_message_right_lib/1 -> BusAssignment_Std_ID423/1
  BusAssignment_Std_ID423/1 -> Out Bus Element1/1
  In Bus Element2/1 -> controller_status_left_lib/1
  controller_status_left_lib/1 -> BusAssignment_Std_ID1830/1
  BusAssignment_Std_ID1830/1 -> Out Bus Element2/1
  In Bus Element3/1 -> controller_status_right_lib/1
  controller_status_right_lib/1 -> BusAssignment_Std_ID1831/1
  BusAssignment_Std_ID1831/1 -> Out Bus Element3/1
  Status Inport/1 -> Status Bus Selector/1
  Status Bus Selector/1 -> BusAssignment_Std_ID422/2  "<ID422>"
  Status Bus Selector/2 -> BusAssignment_Std_ID423/2  "<ID423>"
  Status Bus Selector/3 -> BusAssignment_Std_ID1830/2  "<ID1830>"
  Status Bus Selector/4 -> BusAssignment_Std_ID1831/2  "<ID1831>"

== system AMR_main_24a_TesteMobotic/CAN DB Parser Read 7/ReadSubsystem ==
  CANRead_Std : speedgoatlib_IO60X_IO69X/CAN/CAN Read   moduleType=IO691  id=1  channel=1  canType=CAN (HS)  messageType=CAN (HS)  useBusOut=on  HasMulRead=Specify by IDs  MsgIDlist=[1459]  isEFF=off  LabelInHex=off  enableInput=off  initValues=[691 1 -1 0 1 1 0 1 2 0 1 1459]  ts=-1
  Data Type ConversionStd : DataTypeConversion  OutDataTypeStr=uint8  SaturateOnIntegerOverflow=off  RndMeth=Floor
  StdSelector_ : Selector  IndexOptions=Index vector (dialog)  Indices=1  OutputSizes=1
  Std_ : Outport  PortName=Raw_Rx  Element=Std.ID1459
  StdStatus_ : Outport  Port=2  PortName=Status_Rx  Element=Std.ID1459
  wires:
  CANRead_Std/1 -> Data Type ConversionStd/1
  CANRead_Std/2 -> Std_/1
  Data Type ConversionStd/1 -> StdSelector_/1
  StdSelector_/1 -> StdStatus_/1

== system AMR_main_24a_TesteMobotic/CAN DB Parser Read 7/UnpackSubsystem ==
  In Bus Element : Inport  PortName=Unpack_In  Element=Std.ID1459
  Status Inport : Inport  Port=2
  BusAssignment_Std_ID1459 : BusAssignment  AssignedSignals=MessageStatus.Status
  Status Bus Selector : BusSelector  OutputSignals=Std.ID1459
  feedback_word_lib : tramontina_database_moboticlib/CAN unpack/feedback_word  SystemSampleTime=-1  VariantActivationTime=update diagram  AllowFlexibleInterface=on  Latency=0  AutoFrameSizeCalculation=off
  Out Bus Element : Outport  PortName=Unpack_Out  Element=ID1459_feedback_word
  wires:
  In Bus Element/1 -> feedback_word_lib/1
  feedback_word_lib/1 -> BusAssignment_Std_ID1459/1
  BusAssignment_Std_ID1459/1 -> Out Bus Element/1
  Status Inport/1 -> Status Bus Selector/1
  Status Bus Selector/1 -> BusAssignment_Std_ID1459/2  "<ID1459>"

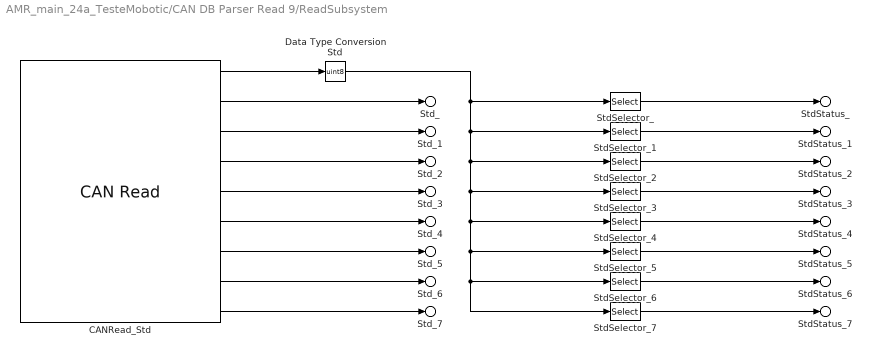
== system AMR_main_24a_TesteMobotic/CAN DB Parser Read 9/ReadSubsystem ==
  CANRead_Std : speedgoatlib_IO60X_IO69X/CAN/CAN Read   moduleType=IO691  id=1  channel=1  canType=CAN (HS)  messageType=CAN (HS)  useBusOut=on  HasMulRead=Specify by IDs  MsgIDlist="[288  343  368  369  370  371  372  373]"  isEFF=off  LabelInHex=off  enableInput=off  initValues=[691 1 -1 0 1 1 0 1 2 0 8 288 343 368 369 370 371 372 373]  ts=-1
  Data Type ConversionStd : DataTypeConversion  OutDataTypeStr=uint8  SaturateOnIntegerOverflow=off  RndMeth=Floor
  StdSelector_ : Selector  IndexOptions=Index vector (dialog)  Indices=1  OutputSizes=1
  StdSelector_1 : Selector  IndexOptions=Index vector (dialog)  Indices=2  OutputSizes=1
  StdSelector_2 : Selector  IndexOptions=Index vector (dialog)  Indices=3  OutputSizes=1
  StdSelector_3 : Selector  IndexOptions=Index vector (dialog)  Indices=4  OutputSizes=1
  StdSelector_4 : Selector  IndexOptions=Index vector (dialog)  Indices=5  OutputSizes=1
  StdSelector_5 : Selector  IndexOptions=Index vector (dialog)  Indices=6  OutputSizes=1
  StdSelector_6 : Selector  IndexOptions=Index vector (dialog)  Indices=7  OutputSizes=1
  StdSelector_7 : Selector  IndexOptions=Index vector (dialog)  Indices=8  OutputSizes=1
  Std_ : Outport  PortName=Raw_Rx  Element=Std.ID288
  Std_1 : Outport  PortName=Raw_Rx  Element=Std.ID343
  Std_2 : Outport  PortName=Raw_Rx  Element=Std.ID368
  Std_3 : Outport  PortName=Raw_Rx  Element=Std.ID369
  Std_4 : Outport  PortName=Raw_Rx  Element=Std.ID370
  Std_5 : Outport  PortName=Raw_Rx  Element=Std.ID371
  Std_6 : Outport  PortName=Raw_Rx  Element=Std.ID372
  Std_7 : Outport  PortName=Raw_Rx  Element=Std.ID373
  StdStatus_ : Outport  Port=2  PortName=Status_Rx  Element=Std.ID288
  StdStatus_1 : Outport  Port=2  PortName=Status_Rx  Element=Std.ID343
  StdStatus_2 : Outport  Port=2  PortName=Status_Rx  Element=Std.ID368
  StdStatus_3 : Outport  Port=2  PortName=Status_Rx  Element=Std.ID369
  StdStatus_4 : Outport  Port=2  PortName=Status_Rx  Element=Std.ID370
  StdStatus_5 : Outport  Port=2  PortName=Status_Rx  Element=Std.ID371
  StdStatus_6 : Outport  Port=2  PortName=Status_Rx  Element=Std.ID372
  StdStatus_7 : Outport  Port=2  PortName=Status_Rx  Element=Std.ID373
  wires:
  CANRead_Std/1 -> Data Type ConversionStd/1
  CANRead_Std/2 -> Std_/1
  CANRead_Std/3 -> Std_1/1
  CANRead_Std/4 -> Std_2/1
  CANRead_Std/5 -> Std_3/1
  CANRead_Std/6 -> Std_4/1
  CANRead_Std/7 -> Std_5/1
  CANRead_Std/8 -> Std_6/1
  CANRead_Std/9 -> Std_7/1
  Data Type ConversionStd/1 -> StdSelector_6/1, StdSelector_7/1, StdSelector_5/1, StdSelector_4/1, StdSelector_3/1, StdSelector_2/1, StdSelector_1/1, StdSelector_/1
  StdSelector_/1 -> StdStatus_/1
  StdSelector_1/1 -> StdStatus_1/1
  StdSelector_2/1 -> StdStatus_2/1
  StdSelector_3/1 -> StdStatus_3/1
  StdSelector_4/1 -> StdStatus_4/1
  StdSelector_5/1 -> StdStatus_5/1
  StdSelector_6/1 -> StdStatus_6/1
  StdSelector_7/1 -> StdStatus_7/1

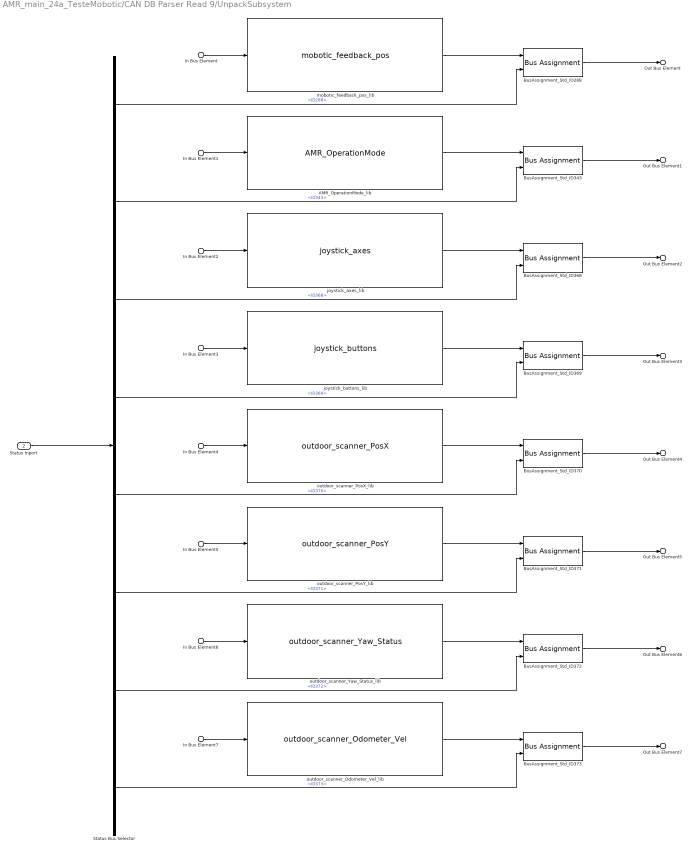
== system AMR_main_24a_TesteMobotic/CAN DB Parser Read 9/UnpackSubsystem ==
  In Bus Element : Inport  PortName=Unpack_In  Element=Std.ID288
  In Bus Element1 : Inport  PortName=Unpack_In  Element=Std.ID343
  In Bus Element2 : Inport  PortName=Unpack_In  Element=Std.ID368
  In Bus Element3 : Inport  PortName=Unpack_In  Element=Std.ID369
  In Bus Element4 : Inport  PortName=Unpack_In  Element=Std.ID370
  In Bus Element5 : Inport  PortName=Unpack_In  Element=Std.ID371
  In Bus Element6 : Inport  PortName=Unpack_In  Element=Std.ID372
  In Bus Element7 : Inport  PortName=Unpack_In  Element=Std.ID373
  Status Inport : Inport  Port=2
  AMR_OperationMode_lib : tramontina_database_nvidialib/CAN unpack/AMR_OperationMode  SystemSampleTime=-1  VariantActivationTime=update diagram  AllowFlexibleInterface=on  Latency=0  AutoFrameSizeCalculation=off
  BusAssignment_Std_ID{288,343,368..373} (8 alike) : BusAssignment  AssignedSignals=MessageStatus.Status
  Status Bus Selector : BusSelector  OutputSignals=Std.ID288,Std.ID343,Std.ID368,Std.ID369,Std.ID370,Std.ID371,Std.ID372,Std.ID373
  joystick_axes_lib : tramontina_database_nvidialib/CAN unpack/joystick_axes  SystemSampleTime=-1  VariantActivationTime=update diagram  AllowFlexibleInterface=on  Latency=0  AutoFrameSizeCalculation=off
  joystick_buttons_lib : tramontina_database_nvidialib/CAN unpack/joystick_buttons  SystemSampleTime=-1  VariantActivationTime=update diagram  AllowFlexibleInterface=on  Latency=0  AutoFrameSizeCalculation=off
  mobotic_feedback_pos_lib : tramontina_database_nvidialib/CAN unpack/mobotic_feedback_pos  SystemSampleTime=-1  VariantActivationTime=update diagram  AllowFlexibleInterface=on  Latency=0  AutoFrameSizeCalculation=off
  outdoor_scanner_Odometer_Vel_lib : tramontina_database_nvidialib/CAN unpack/outdoor_scanner_Odometer_Vel  SystemSampleTime=-1  VariantActivationTime=update diagram  AllowFlexibleInterface=on  Latency=0  AutoFrameSizeCalculation=off
  outdoor_scanner_PosX_lib : tramontina_database_nvidialib/CAN unpack/outdoor_scanner_PosX  SystemSampleTime=-1  VariantActivationTime=update diagram  AllowFlexibleInterface=on  Latency=0  AutoFrameSizeCalculation=off
  outdoor_scanner_PosY_lib : tramontina_database_nvidialib/CAN unpack/outdoor_scanner_PosY  SystemSampleTime=-1  VariantActivationTime=update diagram  AllowFlexibleInterface=on  Latency=0  AutoFrameSizeCalculation=off
  outdoor_scanner_Yaw_Status_lib : tramontina_database_nvidialib/CAN unpack/outdoor_scanner_Yaw_Status  SystemSampleTime=-1  VariantActivationTime=update diagram  AllowFlexibleInterface=on  Latency=0  AutoFrameSizeCalculation=off
  Out Bus Element : Outport  PortName=Unpack_Out  Element=ID288_mobotic_feedback_pos
  Out Bus Element1 : Outport  PortName=Unpack_Out  Element=ID343_AMR_OperationMode
  Out Bus Element2 : Outport  PortName=Unpack_Out  Element=ID368_joystick_axes
  Out Bus Element3 : Outport  PortName=Unpack_Out  Element=ID369_joystick_buttons
  Out Bus Element4 : Outport  PortName=Unpack_Out  Element=ID370_outdoor_scanner_PosX
  Out Bus Element5 : Outport  PortName=Unpack_Out  Element=ID371_outdoor_scanner_PosY
  Out Bus Element6 : Outport  PortName=Unpack_Out  Element=ID372_outdoor_scanner_Yaw_Status
  Out Bus Element7 : Outport  PortName=Unpack_Out  Element=ID373_outdoor_scanner_Odometer_Vel
  wires:
  In Bus Element/1 -> mobotic_feedback_pos_lib/1
  mobotic_feedback_pos_lib/1 -> BusAssignment_Std_ID288/1
  BusAssignment_Std_ID288/1 -> Out Bus Element/1
  In Bus Element1/1 -> AMR_OperationMode_lib/1
  AMR_OperationMode_lib/1 -> BusAssignment_Std_ID343/1
  BusAssignment_Std_ID343/1 -> Out Bus Element1/1
  In Bus Element2/1 -> joystick_axes_lib/1
  joystick_axes_lib/1 -> BusAssignment_Std_ID368/1
  BusAssignment_Std_ID368/1 -> Out Bus Element2/1
  In Bus Element3/1 -> joystick_buttons_lib/1
  joystick_buttons_lib/1 -> BusAssignment_Std_ID369/1
  BusAssignment_Std_ID369/1 -> Out Bus Element3/1
  In Bus Element4/1 -> outdoor_scanner_PosX_lib/1
  outdoor_scanner_PosX_lib/1 -> BusAssignment_Std_ID370/1
  BusAssignment_Std_ID370/1 -> Out Bus Element4/1
  In Bus Element5/1 -> outdoor_scanner_PosY_lib/1
  outdoor_scanner_PosY_lib/1 -> BusAssignment_Std_ID371/1
  BusAssignment_Std_ID371/1 -> Out Bus Element5/1
  In Bus Element6/1 -> outdoor_scanner_Yaw_Status_lib/1
  outdoor_scanner_Yaw_Status_lib/1 -> BusAssignment_Std_ID372/1
  BusAssignment_Std_ID372/1 -> Out Bus Element6/1
  In Bus Element7/1 -> outdoor_scanner_Odometer_Vel_lib/1
  outdoor_scanner_Odometer_Vel_lib/1 -> BusAssignment_Std_ID373/1
  BusAssignment_Std_ID373/1 -> Out Bus Element7/1
  Status Inport/1 -> Status Bus Selector/1
  Status Bus Selector/1 -> BusAssignment_Std_ID288/2  "<ID288>"
  Status Bus Selector/2 -> BusAssignment_Std_ID343/2  "<ID343>"
  Status Bus Selector/3 -> BusAssignment_Std_ID368/2  "<ID368>"
  Status Bus Selector/4 -> BusAssignment_Std_ID369/2  "<ID369>"
  Status Bus Selector/5 -> BusAssignment_Std_ID370/2  "<ID370>"
  Status Bus Selector/6 -> BusAssignment_Std_ID371/2  "<ID371>"
  Status Bus Selector/7 -> BusAssignment_Std_ID372/2  "<ID372>"
  Status Bus Selector/8 -> BusAssignment_Std_ID373/2  "<ID373>"

== system AMR_main_24a_TesteMobotic/CAN DB Parser Write /BusMapping ==
  AMR_auto_mode : Inport  PortName=InBus  Element=AMR_auto_mode
  AMR_idle_mode : Inport  PortName=InBus  Element=AMR_idle_mode
  AMR_manual_mode : Inport  PortName=InBus  Element=AMR_manual_mode
  ID344_AMR_OperationMode_feedback.OperationMode_auto : Outport  PortName=OutBus  Element=ID344_AMR_OperationMode_feedback.OperationMode_auto
  ID344_AMR_OperationMode_feedback.OperationMode_idle : Outport  PortName=OutBus  Element=ID344_AMR_OperationMode_feedback.OperationMode_idle
  ID344_AMR_OperationMode_feedback.OperationMode_manual : Outport  PortName=OutBus  Element=ID344_AMR_OperationMode_feedback.OperationMode_manual
  wires:
  AMR_auto_mode/1 -> ID344_AMR_OperationMode_feedback.OperationMode_auto/1
  AMR_idle_mode/1 -> ID344_AMR_OperationMode_feedback.OperationMode_idle/1
  AMR_manual_mode/1 -> ID344_AMR_OperationMode_feedback.OperationMode_manual/1

== system AMR_main_24a_TesteMobotic/CAN DB Parser Write /Convert2BusArray ==
  In1 : Inport  PortName=InBus  Element=ID344_AMR_OperationMode_feedback
  BusArray : Concatenate  NumInputs=1
  BusArrayOut : Outport
  wires:
  In1/1 -> BusArray/1
  BusArray/1 -> BusArrayOut/1

== system AMR_main_24a_TesteMobotic/CAN DB Parser Write /PackSubsystem ==
  In Bus Element : Inport  PortName=PackIn  Element=ID344_AMR_OperationMode_feedback
  AMR_OperationMode_feedback_lib : tramontina_database_nvidialib/CAN pack/AMR_OperationMode_feedback  SystemSampleTime=-1  VariantActivationTime=update diagram  AllowFlexibleInterface=on  Latency=0  AutoFrameSizeCalculation=off
  In Bus Element1 : Outport  PortName=PackOut  Element=ID344_AMR_OperationMode_feedback
  wires:
  In Bus Element/1 -> AMR_OperationMode_feedback_lib/1
  AMR_OperationMode_feedback_lib/1 -> In Bus Element1/1

== system AMR_main_24a_TesteMobotic/CAN DB Parser Write 1/Convert2BusArray ==
  In1 : Inport  PortName=InBus  Element=ID290_AMR_vehicle_speed
  BusArray : Concatenate  NumInputs=1
  BusArrayOut : Outport
  wires:
  In1/1 -> BusArray/1
  BusArray/1 -> BusArrayOut/1

== system AMR_main_24a_TesteMobotic/CAN DB Parser Write 1/InputSubsystem ==
  In1_1 : Inport
  In1_2 : Inport  Port=2
  ID290_AMR_vehicle_speed.speed_m_per_min : Outport  PortName=OutBus  Element=ID290_AMR_vehicle_speed.speed_m_per_min
  ID290_AMR_vehicle_speed.speed_m_per_s : Outport  PortName=OutBus  Element=ID290_AMR_vehicle_speed.speed_m_per_s
  wires:
  In1_1/1 -> ID290_AMR_vehicle_speed.speed_m_per_min/1
  In1_2/1 -> ID290_AMR_vehicle_speed.speed_m_per_s/1

== system AMR_main_24a_TesteMobotic/CAN DB Parser Write 1/PackSubsystem ==
  In Bus Element : Inport  PortName=PackIn  Element=ID290_AMR_vehicle_speed
  AMR_vehicle_speed_lib : tramontina_database_nvidialib/CAN pack/AMR_vehicle_speed  SystemSampleTime=-1  VariantActivationTime=update diagram  AllowFlexibleInterface=on  Latency=0  AutoFrameSizeCalculation=off
  In Bus Element1 : Outport  PortName=PackOut  Element=ID290_AMR_vehicle_speed
  wires:
  In Bus Element/1 -> AMR_vehicle_speed_lib/1
  AMR_vehicle_speed_lib/1 -> In Bus Element1/1

== system AMR_main_24a_TesteMobotic/CAN DB Parser Write 2/BusMapping ==
  signal1 : Inport  PortName=InBus  Element=signal1
  signal2 : Inport  PortName=InBus  Element=signal2
  ID550_curtis_input_message_left.rpm_set_left : Outport  PortName=OutBus  Element=ID550_curtis_input_message_left.rpm_set_left
  ID551_curtis_input_message_right.rpm_set_right : Outport  PortName=OutBus  Element=ID551_curtis_input_message_right.rpm_set_right
  wires:
  signal1/1 -> ID550_curtis_input_message_left.rpm_set_left/1
  signal2/1 -> ID551_curtis_input_message_right.rpm_set_right/1

== system AMR_main_24a_TesteMobotic/CAN DB Parser Write 2/Convert2BusArray ==
  In1 : Inport  PortName=InBus  Element=ID550_curtis_input_message_left
  In2 : Inport  PortName=InBus  Element=ID551_curtis_input_message_right
  BusArray : Concatenate
  BusArrayOut : Outport
  wires:
  In1/1 -> BusArray/1
  In2/1 -> BusArray/2
  BusArray/1 -> BusArrayOut/1

== system AMR_main_24a_TesteMobotic/CAN DB Parser Write 2/PackSubsystem ==
  In Bus Element : Inport  PortName=PackIn  Element=ID550_curtis_input_message_left
  In Bus Element2 : Inport  PortName=PackIn  Element=ID551_curtis_input_message_right
  curtis_input_message_left_lib : tramontina_database_curtislib/CAN pack/curtis_input_message_left  SystemSampleTime=-1  VariantActivationTime=update diagram  AllowFlexibleInterface=on  Latency=0  AutoFrameSizeCalculation=off
  curtis_input_message_right_lib : tramontina_database_curtislib/CAN pack/curtis_input_message_right  SystemSampleTime=-1  VariantActivationTime=update diagram  AllowFlexibleInterface=on  Latency=0  AutoFrameSizeCalculation=off
  In Bus Element1 : Outport  PortName=PackOut  Element=ID550_curtis_input_message_left
  In Bus Element3 : Outport  PortName=PackOut  Element=ID551_curtis_input_message_right
  wires:
  In Bus Element/1 -> curtis_input_message_left_lib/1
  curtis_input_message_left_lib/1 -> In Bus Element1/1
  In Bus Element2/1 -> curtis_input_message_right_lib/1
  curtis_input_message_right_lib/1 -> In Bus Element3/1

== system AMR_main_24a_TesteMobotic/CAN DB Parser Write 3/Convert2BusArray ==
  In1 : Inport  PortName=InBus  Element=ID0_curtis_input_operational
  BusArray : Concatenate  NumInputs=1
  BusArrayOut : Outport
  wires:
  In1/1 -> BusArray/1
  BusArray/1 -> BusArrayOut/1

== system AMR_main_24a_TesteMobotic/CAN DB Parser Write 3/InputSubsystem ==
  In1_1 : Inport
  ID0_curtis_input_operational.pre_operational : Outport  PortName=OutBus  Element=ID0_curtis_input_operational.pre_operational
  wires:
  In1_1/1 -> ID0_curtis_input_operational.pre_operational/1

== system AMR_main_24a_TesteMobotic/CAN DB Parser Write 3/PackSubsystem ==
  In Bus Element : Inport  PortName=PackIn  Element=ID0_curtis_input_operational
  curtis_input_operational_lib : tramontina_database_curtislib/CAN pack/curtis_input_operational  SystemSampleTime=-1  VariantActivationTime=update diagram  AllowFlexibleInterface=on  Latency=0  AutoFrameSizeCalculation=off
  In Bus Element1 : Outport  PortName=PackOut  Element=ID0_curtis_input_operational
  wires:
  In Bus Element/1 -> curtis_input_operational_lib/1
  curtis_input_operational_lib/1 -> In Bus Element1/1

== system AMR_main_24a_TesteMobotic/CAN DB Parser Write 5/Convert2BusArray ==
  In1 : Inport  PortName=InBus  Element=ID289_mobotic_error_flag
  BusArray : Concatenate  NumInputs=1
  BusArrayOut : Outport
  wires:
  In1/1 -> BusArray/1
  BusArray/1 -> BusArrayOut/1

== system AMR_main_24a_TesteMobotic/CAN DB Parser Write 5/InputSubsystem ==
  In1_1 : Inport
  ID289_mobotic_error_flag.steering_unit_error : Outport  PortName=OutBus  Element=ID289_mobotic_error_flag.steering_unit_error
  wires:
  In1_1/1 -> ID289_mobotic_error_flag.steering_unit_error/1

== system AMR_main_24a_TesteMobotic/CAN DB Parser Write 5/PackSubsystem ==
  In Bus Element : Inport  PortName=PackIn  Element=ID289_mobotic_error_flag
  mobotic_error_flag_lib : tramontina_database_nvidialib/CAN pack/mobotic_error_flag  SystemSampleTime=-1  VariantActivationTime=update diagram  AllowFlexibleInterface=on  Latency=0  AutoFrameSizeCalculation=off
  In Bus Element1 : Outport  PortName=PackOut  Element=ID289_mobotic_error_flag
  wires:
  In Bus Element/1 -> mobotic_error_flag_lib/1
  mobotic_error_flag_lib/1 -> In Bus Element1/1

== system AMR_main_24a_TesteMobotic/CAN DB Parser Write 6/Convert2BusArray ==
  In1 : Inport  PortName=InBus  Element=ID1587_control_word
  BusArray : Concatenate  NumInputs=1
  BusArrayOut : Outport
  wires:
  In1/1 -> BusArray/1
  BusArray/1 -> BusArrayOut/1
